simulink subsystem "closed_loop_kin_mpc_pdplus_control_refsys"  (R2022b)
settings: Solver=VariableStepAuto  StartTime=0.0  StopTime=10.0  RelTol=1e-3
settings Model: Creator=emu  LastModifiedBy=emu

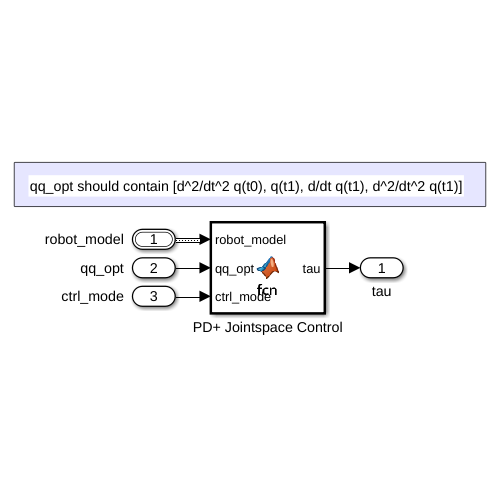
[thumbnail: Simulink's stored preview of the top-level diagram]
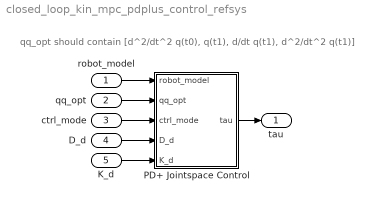
== system closed_loop_kin_mpc_pdplus_control_refsys ==
  note: qq_opt should contain [d^2/dt^2 q(t0), q(t1), d/dt q(t1), d^2/dt^2 q(t1)]
  robot_model : Inport  OutDataTypeStr=Bus: robot_model
  qq_opt : Inport  Port=2
  ctrl_mode : Inport  Port=3
  D_d : Inport  Port=4
  K_d : Inport  Port=5
  PD+ Jointspace Control : MATLAB Function  TreatAsAtomicUnit=on
  tau : Outport
  wires:
  ctrl_mode/1 -> PD+ Jointspace Control/3(ctrl_mode)
  robot_model/1 -> PD+ Jointspace Control/1(robot_model)
  qq_opt/1 -> PD+ Jointspace Control/2(qq_opt)
  PD+ Jointspace Control/1(tau) -> tau/1
  D_d/1 -> PD+ Jointspace Control/4(D_d)
  K_d/1 -> PD+ Jointspace Control/5(K_d)

== matlab function closed_loop_kin_mpc_pdplus_control_refsys/PD+ Jointspace Control ==
  data: robot_model input Bus: robot_model; tau output; qq_opt input; ctrl_mode input; D_d input; K_d input; param_robot parameter
function tau  = fcn(robot_model, qq_opt, ctrl_mode, D_d, K_d, param_robot)

n = param_robot.n_DOF;

if size(qq_opt, 2) ~= 0 && size(qq_opt, 1) ~= 1
    n_red = param_robot.n_red;
    n_indices = param_robot.n_indices;
    q = robot_model.q;
    q_p = robot_model.q_p;
    q_d_pp = qq_opt(1:n_red);
    M = robot_model.M;      % inertia matrix
    g = robot_model.g;
    C = robot_model.C;
    C_rnea = robot_model.C_rnea; % C_rnea(q, q_p) = C(q, q_p)q_p + g(q) = n(q, q_p)

    if(ctrl_mode == 1)
        % Hat den Vorteil, dass hier P und D Terme gewählt werden können!
        q_d_1 = qq_opt(1+n_red:2*n_red);
        q_d_p_1 = qq_opt(1+2*n_red:3*n_red);
        q_d_pp_1 = qq_opt(1+3*n_red:4*n_red);
    
        q_1 = param_robot.q_0_ref';
        q_p_1 = zeros(n,1);
        q_pp_1 = zeros(n,1);
        
        q_1(n_indices) = q_d_1;
        q_p_1(n_indices) = q_d_p_1;
        q_pp_1(n_indices) = q_d_pp_1;
    
        %CT: 
        tau = M * (q_pp_1 - D_d * (q_p - q_p_1) - K_d * (q - q_1)) + C_rnea - g;

        %PD+:
        %tau = M * q_pp_1 + C * q_p_1 - D_d * (q_p - q_p_1) - K_d * (q - q_1);
    else
        q_pp = zeros(n,1);
        q_pp(n_indices) = q_d_pp;
        
        tau = M*q_pp + C_rnea - g;
    end
else
    tau = zeros(n,1);
end
